simulink model "scenario_2"  (R2016b)
settings: Solver=VariableStepAuto  StartTime=0.0  StopTime=1000  FixedStep=0.2  RelTol=1e-3
libraries: simulink x2, fuzblock x1
settings Model: Creator=Administrator  LastModifiedBy=Administrator
settings DataIOCC: LimitDataPoints=on  SaveOutput=off  SaveTime=off
settings OptimizationCC: BlockReduction=off  BooleanDataType=off  LifeSpan=inf
settings DebuggingCC: SaveWithParameterizedLinksMsg=none  UnderspecifiedInitializationDetection=Classic  MergeDetectMultiDrivingBlocksExec=none  SignalResolutionControl=TryResolveAllWithWarning  AllowSymbolicDim=off  SFUnexpectedBacktrackingDiag=warning  SFNoUnconditionalDefaultTransitionDiag=warning  SFExecutionAtInitializationDiag=none
settings HardwareCC: TargetUnknown=on
settings GRTTargetCC: TargetLangStandard=C89/C90 (ANSI)  GeneratePreprocessorConditionals=Disable all

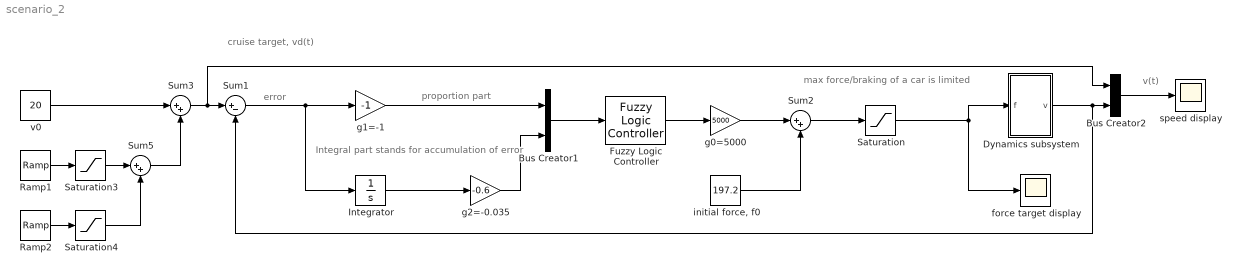
== system scenario_2 ==
  note: max force/braking of a car is limited
  note: error
  note: v(t)
  note: cruise target, vd(t)
  note: proportion part
  note: Integral part stands for accumulation of error
  Bus Creator1 : BusCreator  Inputs=2
  Bus Creator2 : BusCreator  Inputs=2
  Dynamics subsystem : Subsystem
  Fuzzy Logic Controller : fuzblock/Fuzzy Logic  Controller  fis='autoControl.fis'
  Integrator : Integrator
  Ramp1 : simulink/Sources/Ramp  slope=0.2  start=100  X0=0
  Ramp2 : simulink/Sources/Ramp  slope=-0.2  start=500  X0=0
  Saturation : Saturate  UpperLimit=2000  LowerLimit=-2000
  Saturation3 : Saturate  UpperLimit=50  LowerLimit=0
  Saturation4 : Saturate  UpperLimit=0  LowerLimit=-70
  Sum1 : Sum  Inputs=|+-
  Sum2 : Sum  Inputs=|++
  Sum3 : Sum  Inputs=|++
  Sum5 : Sum  Inputs=|++
  force target display : Scope
  g0=5000 : Gain  Gain=5000
  g1=-1 : Gain  Gain=-1
  g2=-0.035 : Gain  Gain=-0.6
  "initial force, f0" : Constant  Value=197.2
  speed display : Scope
  v0 : Constant  Value=20
  wires:
  Saturation/1 -> Dynamics subsystem/1(f), force target display/1
  Sum1/1 -> Integrator/1, g1=-1/1
  Integrator/1 -> g2=-0.035/1
  g1=-1/1 -> Bus Creator1/1
  g2=-0.035/1 -> Bus Creator1/2
  Bus Creator1/1 -> Fuzzy Logic Controller/1
  Fuzzy Logic Controller/1 -> g0=5000/1
  Bus Creator2/1 -> speed display/1
  Dynamics subsystem/1(v) -> Bus Creator2/2, Sum1/2
  g0=5000/1 -> Sum2/1
  Sum2/1 -> Saturation/1
  "initial force, f0"/1 -> Sum2/2
  Ramp1/1 -> Saturation3/1
  Saturation3/1 -> Sum5/1
  Ramp2/1 -> Saturation4/1
  Saturation4/1 -> Sum5/2
  Sum3/1 -> Bus Creator2/1, Sum1/1
  v0/1 -> Sum3/1
  Sum5/1 -> Sum3/2

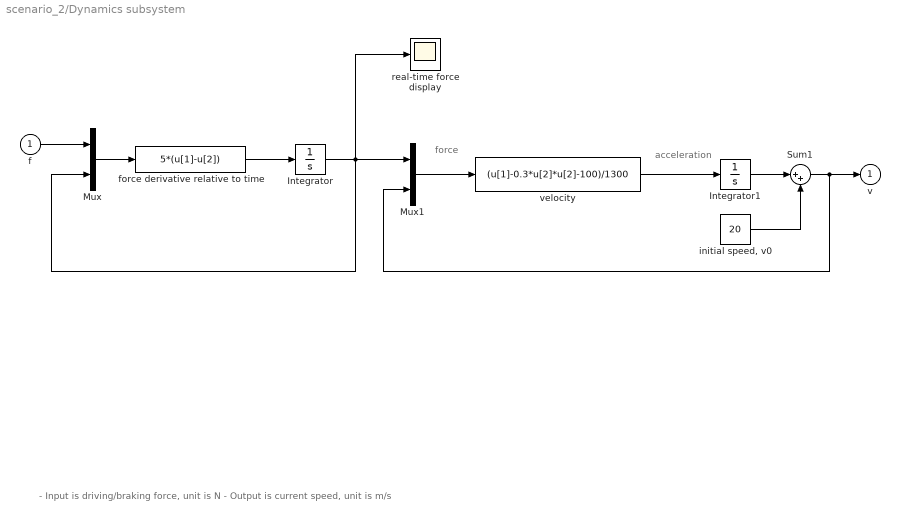
== system scenario_2/Dynamics subsystem ==
  note: - Input is driving/braking force, unit is N
      | - Output is current speed, unit is m/s
  note: acceleration
  note: force
  f : Inport
  Integrator : Integrator
  Integrator1 : Integrator
  Mux : Mux  Inputs=2
  Mux1 : Mux  Inputs=2
  Sum1 : Sum  Inputs=|++
  force derivative relative to time : Fcn  Expr=5*(u[1]-u[2])
  "initial speed, v0" : Constant  Value=20
  real-time force display : Scope
  velocity : Fcn  Expr=(u[1]-0.3*u[2]*u[2]-100)/1300
  v : Outport  InitialOutput=0
  wires:
  f/1 -> Mux/1
  Integrator1/1 -> Sum1/1
  "initial speed, v0"/1 -> Sum1/2
  Integrator/1 -> real-time force display/1, Mux1/1, Mux/2
  Mux/1 -> force derivative relative to time/1
  force derivative relative to time/1 -> Integrator/1
  Sum1/1 -> v/1, Mux1/2
  Mux1/1 -> velocity/1
  velocity/1 -> Integrator1/1
